simulink model "rtwdemo_tflcustomentry"  (Simulink 7.6)
settings: Solver=ode3  StartTime=0.0  StopTime=20  FixedStep=.01  RelTol=1e-3  SampleTimeConstraint=Specified
PreLoadFcn:
  | addpath(fullfile(matlabroot,'toolbox','rtw','rtwdemos','tfl_demo'));
  | sl_refresh_customizations;
libraries: rtwdemowidgets x2
Description:
  | TFL custom entry replacement.
  | This model demonstrates how to use TFL custom entries to create
  | your own matching function and to modify the matched entry by
  | injecting constants as additional implementation arguments.
settings Model: Creator=The MathWorks Inc.  ExtModeAutoUpdateStatusClock=off
settings MATStruct: SampleTime=1  Offset=0  Priority=[30.0]
settings DataIOCC: SaveOutput=off  SaveTime=off  SignalLoggingName=sigsOut
settings OptimizationCC: InlineParams=on  UseIntDivNetSlope=on  InlineInvariantSignals=on  EnhancedBackFolding=on  BooleansAsBitfields=on  PassReuseOutputArgsAs=Individual arguments  StateBitsets=on  DataBitsets=on  UseTempVars=on  ZeroExternalMemoryAtStartup=off  ZeroInternalMemoryAtStartup=off  NoFixptDivByZeroProtection=on  EfficientFloat2IntCast=on  OptimizeModelRefInitCode=on  LifeSpan=1
settings DebuggingCC: CheckExecutionContextPreStartOutputMsg=on  CheckExecutionContextRuntimeOutputMsg=on  SolverPrmCheckMsg=none  IntegerOverflowMsg=none  ParameterPrecisionLossMsg=none  StrictBusMsg=ErrorOnBusTreatedAsVector
settings HardwareCC: ProdBitPerLong=64  ProdIntDivRoundTo=Zero  ProdEndianess=LittleEndian  ProdWordSize=64  ProdHWDeviceType=Specified  TargetHWDeviceType=32-bit Generic
settings SFSimCC: SFSimEnableDebug=off  SFSimOverflowDetection=off  SimParseCustomCode=off
settings RTWCC: SystemTargetFile=ert.tlc  GenCodeOnly=on  TemplateMakefile=ert_default_tmf  Description=Real-Time Workshop Embedded Coder  GenerateReport=on  RTWVerbose=off  ProcessScript=ert_make_rtw_hook  IncludeHyperlinkInReport=on  LaunchReport=on  GenerateTraceInfo=on  GenerateTraceReport=on  GenerateTraceReportSl=on  GenerateTraceReportSf=on  GenerateTraceReportEml=on
settings CodeAppCC: ForceParamTrailComments=on  IgnoreCustomStorageClasses=off  IgnoreTestpoints=on  SimulinkDataObjDesc=on  CustomSymbolStrGlobalVar=rt$N$M  CustomSymbolStrType=$N$M  CustomSymbolStrFcn=$N$M$F  CustomSymbolStrMacro=$N$M  InsertBlockDesc=on
settings ERTTargetCC: TargetFunctionLibrary=Custom TFL Entry Examples  MultiwordLength=2048  GenerateSampleERTMain=on  IncludeMdlTerminateFcn=off  SupportNonFinite=off  SupportComplex=off  InlinedParameterPlacement=NonHierarchical  ERTCustomFileTemplate=example_file_process.tlc  ConvertIfToSwitch=off

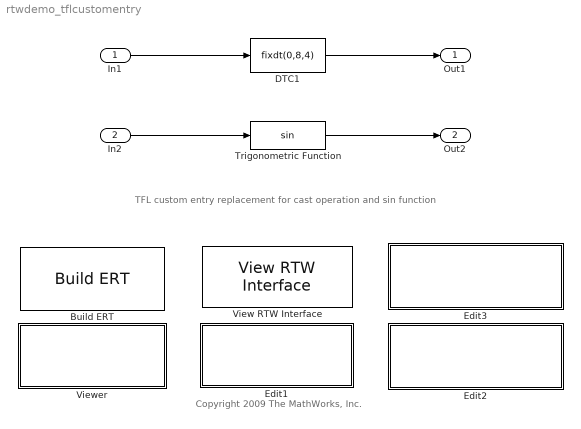
== system rtwdemo_tflcustomentry ==
  note: Copyright 2009 The MathWorks, Inc.
  note: TFL custom entry replacement for cast operation and sin function
  In1 : Inport  OutDataTypeStr=fixdt(0,16,2)  PortDimensions=1  SampleTime=1
  In2 : Inport  Port=2  OutDataTypeStr=double  PortDimensions=1  SampleTime=1
  Build ERT : rtwdemowidgets/Build ERT  SystemSampleTime=-1  attrib_overrides={'GenFloatMathFcnCalls'}
  DTC1 : DataTypeConversion  OutDataTypeStr=fixdt(0,8,4)  SaturateOnIntegerOverflow=on  RndMeth=Zero
  Edit1 : Subsystem  mask{attrib_overrides={}}
      mask prompts: attrib_overrides "List of attributes to preserve (cell of strings):"
      mask help: Enter the attributes of the configuration set that you want preserved. Otherwise, the default configuration script will override your current settings.
      settings: OpenFcn=edit('tfl_table_customentry');
      mask Display:
      | disp(['View/edit TFL \n', ...
      |          'Definition File \n (double-click)'])
  Edit2 : Subsystem  mask{attrib_overrides={}}
      mask prompts: attrib_overrides "List of attributes to preserve (cell of strings):"
      mask help: Enter the attributes of the configuration set that you want preserved. Otherwise, the default configuration script will override your current settings.
      settings: OpenFcn=edit(fullfile(matlabroot,'toolbox','rtw','rtwdemos','tfl_demo', 'sl_customization.m'));
      mask Display:
      | disp(['View/edit TFL Registration\n',...
      | 	  'sl_customization.m\n(double-click)'])
  Edit3 : Subsystem  mask{attrib_overrides={}}
      mask prompts: attrib_overrides "List of attributes to preserve (cell of strings):"
      mask help: Enter the attributes of the configuration set that you want preserved. Otherwise, the default configuration script will override your current settings.
      settings: OpenFcn=|
      | edit(fullfile(matlabroot,'toolbox','rtw','rtwdemos','tfl_demo', '+CustomTflEntry', '@TflCustomCastEntry', 'TflCustomCastEntry.m'));
      | edit(fullfile(matlabroot,'toolbox','rtw','rtwdemos','tfl_demo', '+CustomTflEntry', '@TflCustomFunctionEntry', 'TflCustomFunctionEntry.m'));
      mask Display:
      | disp(['View/edit custom\n',...
      | 	  'entry definition\n(double-click)'])
  Trigonometric Function : Trigonometry
  View RTW Interface : rtwdemowidgets/View RTW Interface  SystemSampleTime=-1
  Viewer : Subsystem  mask{attrib_overrides={}}
      mask prompts: attrib_overrides "List of attributes to preserve (cell of strings):"
      mask help: Enter the attributes of the configuration set that you want preserved. Otherwise, the default configuration script will override your current settings.
      settings: OpenFcn=|
      | tfl = tfl_table_customentry;
      | obj = RTW.viewTfl(tfl);
      | clear tfl obj;
      mask Display:
      | disp(['Invoke TFL Viewer on\n',...
      | 	  'TFL definition file\n(double-click)'])
  Out1 : Outport
  Out2 : Outport  Port=2
  wires:
  In1/1 -> DTC1/1
  DTC1/1 -> Out1/1
  In2/1 -> Trigonometric Function/1
  Trigonometric Function/1 -> Out2/1

== system rtwdemo_tflcustomentry/Edit1 ==

== system rtwdemo_tflcustomentry/Edit2 ==

== system rtwdemo_tflcustomentry/Edit3 ==

== system rtwdemo_tflcustomentry/Viewer ==
